simulink model "PIDAdjVirtualCAN"  (R2025a)
settings: Solver=FixedStepAuto  StartTime=0.0  StopTime=10  FixedStep=1e-4  RelTol=1e-3
undefined symbols (not defined in the file): canChannel, Data, ID
libraries: canlib x3
settings Model: DataDictionary=System.sldd  Creator=tecnicomcbti  LastModifiedBy=tecnicomcbti
settings SolverCC: ConcurrentTasks=on  AutoInsertRateTranBlk=on
settings DebuggingCC: UnderspecifiedInitializationDetection=Classic  MergeDetectMultiDrivingBlocksExec=none
settings ModelReferenceCC: PropagateSignalLabelsOutOfModel=off

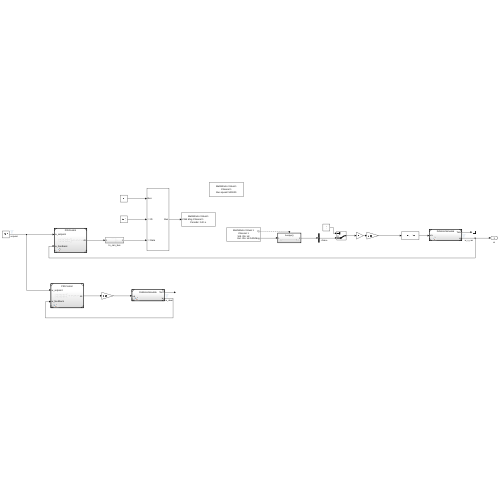
[thumbnail: Simulink's stored preview of the top-level diagram]
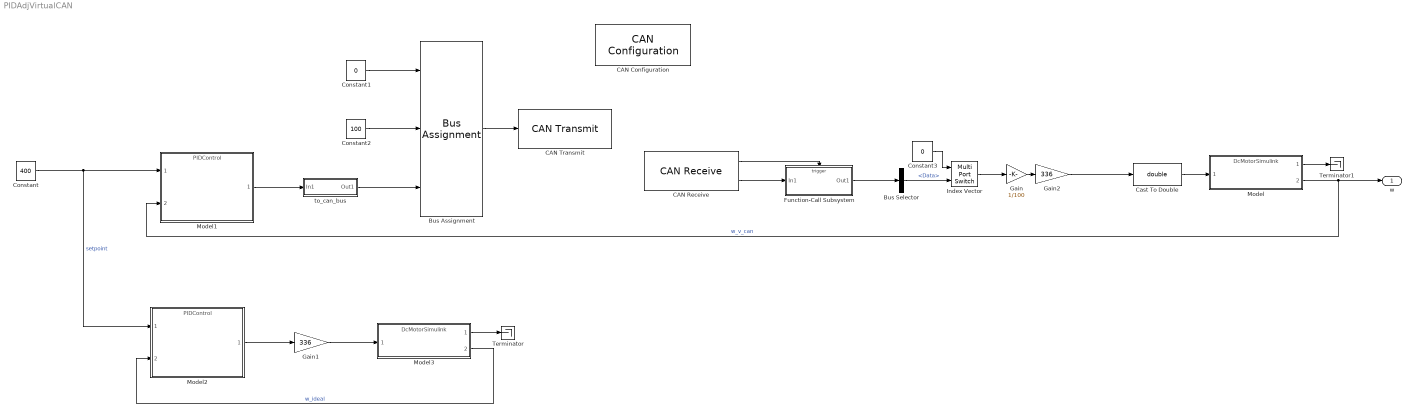
== system PIDAdjVirtualCAN ==
  Bus Assignment : BusAssignment  AssignedSignals=ID,Data
  Bus Selector : BusSelector  OutputSignals=Data
  CAN Configuration : canlib/CAN Configuration  BlockHandle=163.0016  Device=MathWorks Virtual 1 (Channel 1)  DeviceMenu=MathWorks Virtual 1 (Channel 1)  ObjConstructor=canChannel('MathWorks', 'Virtual 1', 1)  BusSpeed=500000  EnableBitParameters=off  AckMode=Normal
  CAN Receive : canlib/CAN Receive  BlockHandle=164.0015  Device=MathWorks Virtual 1 (Channel 1)  DeviceMenu=MathWorks Virtual 1 (Channel 1)  ObjConstructor=canChannel('MathWorks', 'Virtual 1', 1)  EnableStandardIDsFilter=off  StdIDsCombo=Allow all  StandardIDs=0  EnableExtendedIDsFilter=off  ExtIDsCombo=Allow all  ExtendedIDs=0  SampleTime=10e-3  MsgsPerTimestep=1  InternalFilterUpdateStatus=on  BusOutput=on
  CAN Transmit : canlib/CAN Transmit  BlockHandle=167.001  Device=MathWorks Virtual 1 (Channel 1)  DeviceMenu=MathWorks Virtual 1 (Channel 1)  ObjConstructor=canChannel('MathWorks', 'Virtual 1', 1)  EnableEventTransmit=off  EnablePeriodicTransmit=on  MessagePeriod=10e-3
  Cast To Double : DataTypeConversion  OutDataTypeStr=double  SaturateOnIntegerOverflow=off  RndMeth=Floor
  Constant : Constant  Value=400
  Constant1 : Constant  Value=0  OutDataTypeStr=Bus: CAN_MESSAGE_BUS
  Constant2 : Constant  Value=100  OutDataTypeStr=uint32
  Constant3 : Constant  Value=0
  Function-Call Subsystem : Subsystem  TreatAsAtomicUnit=on
  Gain : Gain  Gain=1/100
  Gain1 : Gain  Gain=336
  Gain2 : Gain  Gain=336
  Index Vector : MultiPortSwitch  DataPortOrder=Zero-based contiguous  Inputs=1  zeroidx=on  SaturateOnIntegerOverflow=off  InputSameDT=off
  Model : ModelReference  ModelNameDialog=DcMotorSimulink.slx  SimulationMode=Normal  ModelReferenceVersion=2.10
  Model1 : ModelReference  ModelNameDialog=PIDControl.slx  SimulationMode=Normal  ModelReferenceVersion=1.6
  Model2 : ModelReference  ModelNameDialog=PIDControl.slx  SimulationMode=Normal  ModelReferenceVersion=1.6
  Model3 : ModelReference  ModelNameDialog=DcMotorSimulink.slx  SimulationMode=Normal  ModelReferenceVersion=2.10
  Terminator : Terminator
  Terminator1 : Terminator
  to_can_bus : Subsystem
  w : Outport
  wires:
  Gain/1 -> Gain2/1
  Gain1/1 -> Model3/1
  Model2/1 -> Gain1/1
  Constant3/1 -> Index Vector/1
  Gain2/1 -> Cast To Double/1
  Cast To Double/1 -> Model/1
  Bus Assignment/1 -> CAN Transmit/1
  Constant1/1 -> Bus Assignment/1
  Index Vector/1 -> Gain/1
  Model1/1 -> to_can_bus/1(In1)
  Function-Call Subsystem/1(Out1) -> Bus Selector/1
  CAN Receive/2 -> Function-Call Subsystem/1(In1)
  to_can_bus/1(Out1) -> Bus Assignment/3
  Constant/1 -> Model2/1, Model1/1  "setpoint"
  CAN Receive/1 -> Function-Call Subsystem/Trigger
  Bus Selector/1 -> Index Vector/2  "<Data>"
  Model3/2 -> Model2/2  "w_ideal"
  Constant2/1 -> Bus Assignment/2
  Model3/1 -> Terminator/1
  Model/2 -> Model1/2, w/1  "w_v_can"
  Model/1 -> Terminator1/1

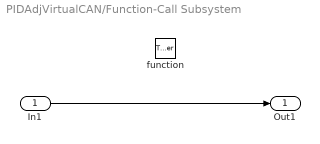
== system PIDAdjVirtualCAN/Function-Call Subsystem ==
  In1 : Inport
  function : TriggerPort  TriggerType=function-call  VariantControl=(inherit)
  Out1 : Outport
  wires:
  In1/1 -> Out1/1

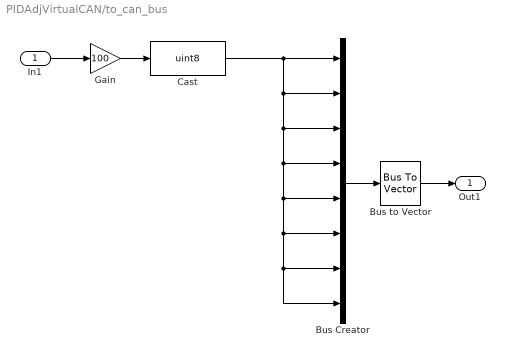
== system PIDAdjVirtualCAN/to_can_bus ==
  In1 : Inport
  Bus Creator : BusCreator  Inputs=8
  Bus to Vector : BusToVector
  Cast : DataTypeConversion  OutDataTypeStr=uint8  SaturateOnIntegerOverflow=off  RndMeth=Floor
  Gain : Gain  Gain=100
  Out1 : Outport
  wires:
  Gain/1 -> Cast/1
  In1/1 -> Gain/1
  Cast/1 -> Bus Creator/8, Bus Creator/7, Bus Creator/6, Bus Creator/5, Bus Creator/4, Bus Creator/3, Bus Creator/2, Bus Creator/1
  Bus Creator/1 -> Bus to Vector/1
  Bus to Vector/1 -> Out1/1
